simulink model "HALLA_Senia_Channel_Noise_Model"  (Simulink 10.1)
settings: Solver=VariableStepAuto  StartTime=0.0  StopTime=10.0  RelTol=1e-3
libraries: commrandsrc3 x2, commchan3 x2, commsink2 x2, commblkcod2 x2
settings Model: Creator=haithem amirouche  LastModifiedBy=acer
settings DataIOCC: SaveFormat=Dataset
settings OptimizationCC: LifeSpan=auto
settings DebuggingCC: UnderspecifiedInitializationDetection=Simplified  MergeDetectMultiDrivingBlocksExec=error  SFUnexpectedBacktrackingDiag=error  SFNoUnconditionalDefaultTransitionDiag=error  SFExecutionAtInitializationDiag=warning
settings HardwareCC: ProdBitPerPointer=64  ProdBitPerSizeT=64  ProdBitPerPtrDiffT=64  ProdLargestAtomicFloat=Float  ProdIntDivRoundTo=Zero  ProdEndianess=LittleEndian  ProdWordSize=64  ProdHWDeviceType=Intel->x86-64 (Windows64)
settings ModelReferenceCC: PropagateSignalLabelsOutOfModel=on
settings GRTTargetCC: TargetLangStandard=C99 (ISO)  CombineOutputUpdateFcns=on  GRTInterface=off
settings ConfigComp: CovMetricSettings=dwe  CovHtmlReporting=off  CovSaveCumulativeToWorkspaceVar=off  CovSaveSingleToWorkspaceVar=off  CovExternalEMLEnable=on

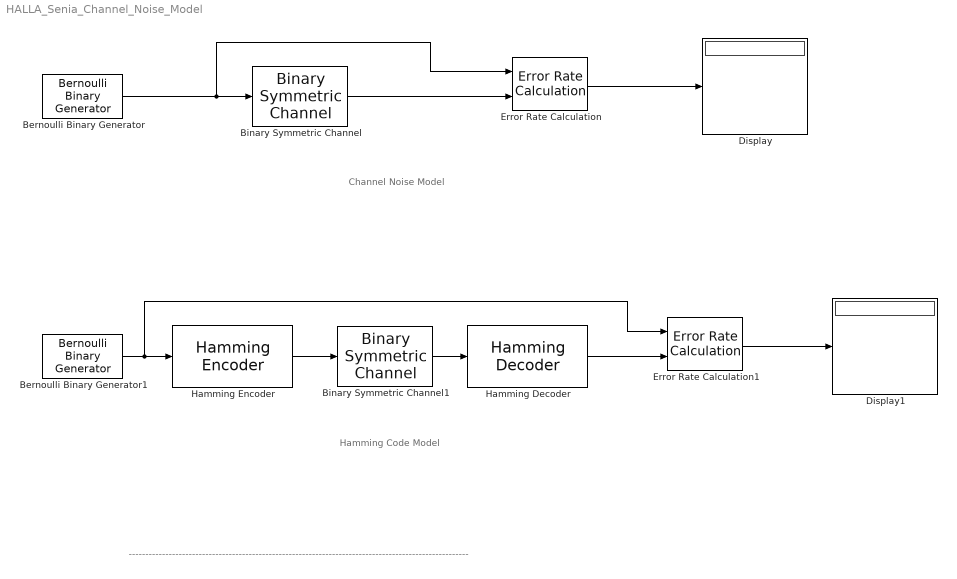
== system HALLA_Senia_Channel_Noise_Model ==
  note: Channel Noise Model
  note: Hamming Code Model
  note: ------------------------------------------------------------------------------------------------------
  Bernoulli Binary Generator : commrandsrc3/Bernoulli Binary Generator  ProbabilityOfZero=0.5  SeedSource=Parameter  Seed=61  SampleTime=1/1200  SamplesPerFrame=1  OutputDataType=double  SimulateUsing=Interpreted execution
  Bernoulli Binary Generator1 : commrandsrc3/Bernoulli Binary Generator  ProbabilityOfZero=0.5  SeedSource=Parameter  Seed=61  SampleTime=1/1200  SamplesPerFrame=4  OutputDataType=double  SimulateUsing=Interpreted execution
  Binary Symmetric Channel : commchan3/Binary Symmetric Channel  ErrorProbability=0.01  ErrorVectorOutputPort=off  OutputDataType=double  OutputDataTypeSL=double  Seed=2137  SimulateUsing=Code generation
      settings: SourceProductBaseCode=CM
  Binary Symmetric Channel1 : commchan3/Binary Symmetric Channel  ErrorProbability=0.01  ErrorVectorOutputPort=off  OutputDataType=double  OutputDataTypeSL=double  Seed=2137  SimulateUsing=Code generation
      settings: SourceProductBaseCode=CM
  Display : Display
  Display1 : Display
  Error Rate Calculation : commsink2/Error Rate Calculation  N=0  st_delay=0  cp_mode=Entire frame  subframe=[]  PMode=Port  WsName=ErrorVec  RsMode2=off  stop=on  numErr=100  maxBits=1e6
  Error Rate Calculation1 : commsink2/Error Rate Calculation  N=0  st_delay=0  cp_mode=Entire frame  subframe=[]  PMode=Port  WsName=ErrorVec  RsMode2=off  stop=on  numErr=100  maxBits=1e6
  Hamming Decoder : commblkcod2/Hamming Decoder  n=7  k=4
      settings: SourceProductBaseCode=CM
  Hamming Encoder : commblkcod2/Hamming Encoder  n=7  k=4
      settings: SourceProductBaseCode=CM
  wires:
  Error Rate Calculation/1 -> Display/1
  Binary Symmetric Channel/1 -> Error Rate Calculation/2
  Bernoulli Binary Generator/1 -> Error Rate Calculation/1, Binary Symmetric Channel/1
  Bernoulli Binary Generator1/1 -> Error Rate Calculation1/1, Hamming Encoder/1
  Hamming Encoder/1 -> Binary Symmetric Channel1/1
  Binary Symmetric Channel1/1 -> Hamming Decoder/1
  Hamming Decoder/1 -> Error Rate Calculation1/2
  Error Rate Calculation1/1 -> Display1/1
